simulink model "BaseEngineController_LS_128"  (Simulink 7.7)
settings: Solver=FixedStepDiscrete  StartTime=0.0  StopTime=10.0  RelTol=1e-3
PreLoadFcn:
  | try, eval([bdroot '_setup']); catch, eval('model_setup', ''); end
InitFcn:
  | try, eval([bdroot '_setup']); catch, eval('model_setup', ''); end
undefined symbols (not defined in the file): ECU565, High, motohawk_build_version, motohawk_trunc_name, motohawk_vardec_config_group, motohawk_vardec_path, True
libraries: MotoHawk_lib x1418, motohawk_control_primitives_lib x183, motohawk_engine_lib x32, simulink x21, motohawk_annotations_lib x9, AutoDoc_lib x8, simulink_extras x4, motohawk_ccp_examples_lib x1, motohawk_control_primitives_motoshare_lib x1
(part 20 of 27)

== system BaseEngineController_LS_128/Foreground/Control/Controller/Run/AC Control/AC Comp Low Pressure ==
  HiThresh : Inport
  LowThresh : Inport  Port=2
  Signal : Inport  Port=3
  Hysteresis : Subsystem
  LT : RelationalOperator  ZeroCross=off  InputSameDT=on
  LT1 : RelationalOperator  Operator=<=  ZeroCross=off  InputSameDT=on
  Threshold : Outport
  wires:
  LT/1 -> Hysteresis/1(Hi)  "AboveHiTarget"
  LT1/1 -> Hysteresis/2(Lo)  "BelowLoTarget"
  Signal/1 -> LT/1, LT1/1
  Hysteresis/1("Out (Lo=0, Hi=1)") -> Threshold/1
  HiThresh/1 -> LT/2
  LowThresh/1 -> LT1/2

== system BaseEngineController_LS_128/Foreground/Control/Controller/Run/AC Control/AC Comp Overspeed ==
  HiThresh : Inport
  LowThresh : Inport  Port=2
  Signal : Inport  Port=3
  Hysteresis : Subsystem
  LT : RelationalOperator  ZeroCross=off  InputSameDT=on
  LT1 : RelationalOperator  Operator=<=  ZeroCross=off  InputSameDT=on
  Threshold : Outport
  wires:
  LT/1 -> Hysteresis/1(Hi)  "AboveHiTarget"
  LT1/1 -> Hysteresis/2(Lo)  "BelowLoTarget"
  Signal/1 -> LT/1, LT1/1
  Hysteresis/1("Out (Lo=0, Hi=1)") -> Threshold/1
  HiThresh/1 -> LT/2
  LowThresh/1 -> LT1/2

== system BaseEngineController_LS_128/Foreground/Control/Controller/Run/AC Control/AC Comp Overspeed1 ==
  HiThresh : Inport
  LowThresh : Inport  Port=2
  Signal : Inport  Port=3
  Hysteresis : Subsystem
  LT : RelationalOperator  ZeroCross=off  InputSameDT=on
  LT1 : RelationalOperator  Operator=<=  ZeroCross=off  InputSameDT=on
  Threshold : Outport
  wires:
  LT/1 -> Hysteresis/1(Hi)  "AboveHiTarget"
  LT1/1 -> Hysteresis/2(Lo)  "BelowLoTarget"
  Signal/1 -> LT/1, LT1/1
  Hysteresis/1("Out (Lo=0, Hi=1)") -> Threshold/1
  HiThresh/1 -> LT/2
  LowThresh/1 -> LT1/2

== system BaseEngineController_LS_128/Foreground/Control/Controller/Run/AC Control/AC Comp Underspeed ==
  HiThresh : Inport
  LowThresh : Inport  Port=2
  Signal : Inport  Port=3
  Hysteresis : Subsystem
  LT : RelationalOperator  ZeroCross=off  InputSameDT=on
  LT1 : RelationalOperator  Operator=<=  ZeroCross=off  InputSameDT=on
  Threshold : Outport
  wires:
  LT/1 -> Hysteresis/1(Hi)  "AboveHiTarget"
  LT1/1 -> Hysteresis/2(Lo)  "BelowLoTarget"
  Signal/1 -> LT/1, LT1/1
  Hysteresis/1("Out (Lo=0, Hi=1)") -> Threshold/1
  HiThresh/1 -> LT/2
  LowThresh/1 -> LT1/2

== system BaseEngineController_LS_128/Foreground/Control/Controller/Run/AC Control/AC Evap Temp Hyst ==
  HiThresh : Inport
  LowThresh : Inport  Port=2
  Signal : Inport  Port=3
  Hysteresis : Subsystem
  LT : RelationalOperator  ZeroCross=off  InputSameDT=on
  LT1 : RelationalOperator  Operator=<=  ZeroCross=off  InputSameDT=on
  Threshold : Outport
  wires:
  LT/1 -> Hysteresis/1(Hi)  "AboveHiTarget"
  LT1/1 -> Hysteresis/2(Lo)  "BelowLoTarget"
  Signal/1 -> LT/1, LT1/1
  Hysteresis/1("Out (Lo=0, Hi=1)") -> Threshold/1
  HiThresh/1 -> LT/2
  LowThresh/1 -> LT1/2

== system BaseEngineController_LS_128/Foreground/Control/Controller/Run/AirFlow Manager/ShutDownTasksComplete Reset ==
  Enable : EnablePort
  Constant : Constant  Value=boolean(1)
  motohawk_data_write : MotoHawk_lib/Data Storage Blocks/motohawk_data_write  source=Lookup By Name  structure=Scalar  operation=Write entire data structure at once  sz_vec=-1  sz_row=3  sz_col=2  typ=boolean  nam='ShutDownTasksComplete'  checkNull=off  write_read_only=off  struct_inst_name='Struct1'  struct_name='MyStruct'
  wires:
  Constant/1 -> motohawk_data_write/1

== system BaseEngineController_LS_128/Foreground/Control/Controller/Run/Base Equiv Ratio/Warm Up Fuel Holdoff ==
  TimeSinceRun : Inport
  WarmuUpTimeRatio : Inport  Port=2
  ECTIdx : Inport  Port=3
  Constant : Constant
  Relational Operator : RelationalOperator  OutDataTypeStr=boolean
  Switch : Switch  Criteria=u2 > Threshold
  motohawk_interpolation_1d : MotoHawk_lib/Lookup Tables/motohawk_interpolation_1d  nam='Warmup_Time_Holdoff'  table_data=[0.1 0.1 0.1 0.1 0.1]  show_more=on  data_type=Inherit from 'Table Data'  storage=NonAdaptive  read_level=1  write_level=1  ovr_cals=on  use_help=on  help='Time before warmup fuel multiplier active'  units='sec'  use_min_max=on  min_val=0  max_val=3  use_precision=on  precision='1.3'  gain=1  offset=0  exp=1  use_links=off  prelookup_block=''  output_name=''  use_mototune_group=off  mototune_group=motohawk_vardec_path(gcb)
  Out1 : Outport
  wires:
  ECTIdx/1 -> motohawk_interpolation_1d/1
  motohawk_interpolation_1d/1 -> Relational Operator/2
  TimeSinceRun/1 -> Relational Operator/1
  Relational Operator/1 -> Switch/2
  WarmuUpTimeRatio/1 -> Switch/1
  Constant/1 -> Switch/3
  Switch/1 -> Out1/1

== system BaseEngineController_LS_128/Foreground/Control/Controller/Run/Boost Control/BoostControl Adapt ==
  Active State : Inport
  ITerm : Inport  Port=2
  Enable : EnablePort
  Abs : Abs  SaturateOnIntegerOverflow=on
  Adapt Boost Table : Subsystem  TreatAsAtomicUnit=on
  BoostControl Enable Delay : Subsystem  TreatAsAtomicUnit=on
  Logical Operator1 : Logic  Inputs=3
  Product0 : Product  SaturateOnIntegerOverflow=on  InputSameDT=on  OutDataTypeStr=Inherit: Same as first input
  Relational Operator : RelationalOperator  Operator=<=  InputSameDT=on
  Saturation (Tunable) : Subsystem  AncestorBlock=motohawk_control_primitives_lib/Saturation (Tunable)  mask(Saturation (Tunable)){prefix='BoostAdaptError', UprLim=1, LwrLim=-1, units='', grp=motohawk_vardec_path(gcb)}
      mask prompts: UprLim "Upper Limit"; LwrLim "Lower Limit"; grp "MotoTune Group String"
      mask help: Saturation block with calibratable min/max values.
      mask Display:
      | patch([0 0 1 1], [0 0.075 0.075 0], [230/255 0/255 0/255])
      | patch([0 0 1 1], [0.025 0.05 0.05 0.025], [150/255 0/255 0/255])
      | patch([0 0 1 1], [0 0.025 0.025 0], [0/255 0/255 0/255])
      | 
      | plot([0 .2 .8 1], [.1 .1 1 1])
  motohawk_calibration2 : MotoHawk_lib/Calibration & Probing Blocks/motohawk_calibration  nam='BoostControlAdaptGain'  val=0.001  storage=Calibration  show_more=on  name_source=Use Parameter  data_type=Inherit from 'Default Value'  read_level=1  write_level=1  ovr_cals=on  view_as=Number  enum_struct={'Disabled', 'Enabled'}  vector_style=Wide Row  use_help_units=off  help="'Gain for updating BaseAirflow table.  This fraction of the error is added to the map every 5ms.'"  units='mult'  use_header_enum=off  row_header_enum={}  col_header_enum={}  use_min_max=off  min_val=-inf  max_val=inf  use_precision=on  precision='1.4'  gain=1  offset=0  exp=1  use_mototune_group=on  mototune_group=motohawk_vardec_path(gcb)
  motohawk_calibration3 : MotoHawk_lib/Calibration & Probing Blocks/motohawk_calibration  nam='BoostControlAdaptDelta'  val=2  storage=Calibration  show_more=on  name_source=Use Parameter  data_type=Inherit from 'Default Value'  read_level=1  write_level=1  ovr_cals=on  view_as=Number  enum_struct={'Disabled', 'Enabled'}  vector_style=Wide Row  use_help_units=on  help='Air PID Iterm must be less than this delta to adapt the BaseAirflow table.'  units='mult'  use_header_enum=off  row_header_enum={}  col_header_enum={}  use_min_max=on  min_val=-inf  max_val=inf  use_precision=off  precision=''  gain=1  offset=0  exp=1  use_mototune_group=on  mototune_group=motohawk_vardec_path(gcb)
  motohawk_calibration4 : MotoHawk_lib/Calibration & Probing Blocks/motohawk_calibration  nam='BoostControlAdaptEnable'  val=false  storage=Calibration  show_more=on  name_source=Use Parameter  data_type=Inherit from 'Default Value'  read_level=1  write_level=1  ovr_cals=on  view_as=Enumeration  enum_struct={'Disabled', 'Enabled'}  vector_style=Wide Row  use_help_units=on  help='Determines whether the BaseAirflow table will be adapted using the air PID Iterm.'  units='bool'  use_header_enum=off  row_header_enum={}  col_header_enum={}  use_min_max=off  min_val=-inf  max_val=inf  use_precision=off  precision=''  gain=1  offset=0  exp=1  use_mototune_group=on  mototune_group=motohawk_vardec_path(gcb)
  motohawk_probe3 : MotoHawk_lib/Calibration & Probing Blocks/motohawk_probe  nam='BoostControlAdaptEnabled'  show_more=on  name_source=Use Parameter  read_level=1  view_as=Enumeration  enum_struct={'Not Enabled', 'Enabled'}  vector_style=Wide Row  use_help_units=on  help=''  units=''  use_header_enum=off  row_header_enum={}  col_header_enum={}  use_precision=off  precision=''  gain=1  offset=0  exp=1  use_mototune_group=on  mototune_group=motohawk_vardec_path(gcb)
  wires:
  Abs/1 -> Relational Operator/1
  motohawk_calibration3/1 -> Relational Operator/2
  motohawk_calibration2/1 -> Product0/2
  Product0/1 -> Saturation (Tunable)/1(In)
  ITerm/1 -> Product0/1, Abs/1
  Relational Operator/1 -> Logical Operator1/3
  BoostControl Enable Delay/1(State_Out) -> Logical Operator1/2
  Logical Operator1/1 -> motohawk_probe3/1, Adapt Boost Table/Enable
  Saturation (Tunable)/1(Out) -> Adapt Boost Table/1(error)
  motohawk_calibration4/1 -> Logical Operator1/1
  Active State/1 -> BoostControl Enable Delay/1(State_In)

== system BaseEngineController_LS_128/Foreground/Control/Controller/Run/Boost Control/Universal PID (Tunable & Scheduled) ==
  Actual : Inport
  SetPoint : Inport  Port=2
  ResetAll : Inport  Port=3
  Constant : Constant  Value=0  OutDataTypeStr=Inherit: Inherit via back propagation
  Constant1 : Constant  Value=0
  PID Gain Select1 : Subsystem
  Saturation : motohawk_control_primitives_lib/Saturation  SystemSampleTime=-1
  Switch : Switch  Threshold=0.5
  Universal PID : motohawk_control_primitives_lib/Universal PID  Description=|  SystemSampleTime=-1  samp_time=.005
      | /* Name: ErrorGain Unit:mult ClassID:VAR StorageID:FLASH Access:RW4+RW3+NA2+NA1 TypeID:UINT4                   
      |    Gain:0.000000001 Min:0.000000000 Max:4.000000000 Format:10.9 UpdateID:REMOTE Help:"This gain is applied to "
      |    "the error term before it is used to calculate the P, I and D terms." VardecSig:6C */                       
      |                                                                                                                
      | /* Name: ITermLowerLim Unit:0 ClassID:VAR StorageID:FLASH Access:RW4+RW3+NA2+NA1 TypeID:SINT2 Gain:0.1         
      |    Min:-3276.8 Max:3276.7 Format:5.1 UpdateID:REMOTE Help:"Lower limit on the I-term value." VardecSig:6C */   
      |                                                                                                                
      | /* Name: ITermUpperLim ClassID:VAR StorageID:FLASH Access:RW4+RW3+NA2+NA1 TypeID:SINT2 Gain:0.1 Min:-3276.8    
      |    Max:3276.7 Format:5.1 UpdateID:REMOTE Help:"Upper limit on I-term value." VardecSig:6C */                   
      |                                                                                                                
      | /* Name: PIDOutLowerLim ClassID:VAR StorageID:FLASH Access:RW4+RW3+NA2+NA1 TypeID:SINT2 Gain:0.1               
      |    Min:-3276.8 Max:3276.7 Format:5.1 UpdateID:REMOTE Help:"Lower limit on PID output." VardecSig:6C */         
      |                                                                                                                
      | /* Name: PIDOutUpperLim ClassID:VAR StorageID:FLASH Access:RW4+RW3+NA2+NA1 TypeID:SINT2 Gain:0.1               
      |    Min:-3276.8 Max:3276.7 Format:3.1 UpdateID:REMOTE Help:"Upper limit on PID output." VardecSig:6C */
  motohawk_calibration2 : MotoHawk_lib/Calibration & Probing Blocks/motohawk_calibration  nam=[prefix 'PIDOutUpperLimit']  val=150  storage=Calibration  show_more=on  name_source=Use Parameter  data_type=Inherit from 'Default Value'  read_level=1  write_level=1  ovr_cals=on  view_as=Number  enum_struct={'Disabled', 'Enabled'}  vector_style=Wide Row  use_help_units=on  help='Upper limit on air min governor PID Output.'  units=units  use_header_enum=off  row_header_enum={}  col_header_enum={}  use_min_max=off  min_val=-inf  max_val=inf  use_precision=off  precision=''  gain=1  offset=0  exp=1  use_mototune_group=on  mototune_group=[group ' | Air PID Config']
  motohawk_calibration5 : MotoHawk_lib/Calibration & Probing Blocks/motohawk_calibration  nam=[prefix 'ErrorGain']  val=0.4  storage=Calibration  show_more=on  name_source=Use Parameter  data_type=Inherit from 'Default Value'  read_level=1  write_level=1  ovr_cals=on  view_as=Number  enum_struct={'Disabled', 'Enabled'}  vector_style=Wide Row  use_help_units=on  help='Error gain for the min governor controller. This gain is applied to the RPM error term before it is used to calculate the P, I and D terms.'  units='mult'  use_header_enum=off  row_header_enum={}  col_header_enum={}  use_min_max=on  min_val=-inf  max_val=inf  use_precision=off  precision=''  gain=1  offset=0  exp=1  use_mototune_group=on  mototune_group=[group ' | Air PID Config']
  motohawk_calibration7 : MotoHawk_lib/Calibration & Probing Blocks/motohawk_calibration  nam=[prefix 'ITermLowerLimit']  val=-3  storage=Calibration  show_more=on  name_source=Use Parameter  data_type=Inherit from 'Default Value'  read_level=1  write_level=1  ovr_cals=on  view_as=Number  enum_struct={'Disabled', 'Enabled'}  vector_style=Wide Row  use_help_units=on  help='Lower limit on Air Min Governor I-term value.'  units=units  use_header_enum=off  row_header_enum={}  col_header_enum={}  use_min_max=on  min_val=-inf  max_val=inf  use_precision=off  precision=''  gain=1  offset=0  exp=1  use_mototune_group=on  mototune_group=[group ' | Air PID Config']
  motohawk_calibration8 : MotoHawk_lib/Calibration & Probing Blocks/motohawk_calibration  nam=[prefix 'ITermUpperLimit']  val=55  storage=Calibration  show_more=on  name_source=Use Parameter  data_type=Inherit from 'Default Value'  read_level=1  write_level=1  ovr_cals=on  view_as=Number  enum_struct={'Disabled', 'Enabled'}  vector_style=Wide Row  use_help_units=on  help='Upper limit on Air Min Governor I-term value.'  units=units  use_header_enum=off  row_header_enum={}  col_header_enum={}  use_min_max=on  min_val=-inf  max_val=inf  use_precision=off  precision=''  gain=1  offset=0  exp=1  use_mototune_group=on  mototune_group=[group ' | Air PID Config']
  motohawk_calibration9 : MotoHawk_lib/Calibration & Probing Blocks/motohawk_calibration  nam=[prefix 'PIDOutLowerLimit']  val=-10  storage=Calibration  show_more=on  name_source=Use Parameter  data_type=Inherit from 'Default Value'  read_level=1  write_level=1  ovr_cals=on  view_as=Number  enum_struct={'Disabled', 'Enabled'}  vector_style=Wide Row  use_help_units=on  help='Lower limit on air min governor PID Output.'  units=units  use_header_enum=off  row_header_enum={}  col_header_enum={}  use_min_max=on  min_val=-inf  max_val=inf  use_precision=off  precision=''  gain=1  offset=0  exp=1  use_mototune_group=on  mototune_group=[group ' | Air PID Config']
  motohawk_prelookup1 : MotoHawk_lib/Lookup Tables/motohawk_prelookup  nam=[prefix 'SpeedError']  breakpoint_data=[-200 -90 -30 0 50 103 140 177 213]  show_more=on  data_type=Inherit from 'Table Data'  storage=Constant  read_level=1  write_level=1  ovr_cals=on  use_help=on  help=''  units=''  use_min_max=off  min_val=-inf  max_val=inf  use_precision=off  precision=''  gain=1  offset=0  exp=1  use_links=off  input_name=''  use_mototune_group=on  mototune_group=motohawk_vardec_path(gcb)
  motohawk_probe1 : MotoHawk_lib/Calibration & Probing Blocks/motohawk_probe  nam=[prefix 'PTerm']  show_more=on  name_source=Use Parameter  read_level=1  view_as=Number  enum_struct={'Disabled', 'Enabled'}  vector_style=Wide Row  use_help_units=on  help='Air min governor P term'  units=''  use_header_enum=off  row_header_enum={}  col_header_enum={}  use_precision=on  precision=''  gain=1  offset=0  exp=1  use_mototune_group=on  mototune_group=motohawk_vardec_path(gcb)
  motohawk_probe2 : MotoHawk_lib/Calibration & Probing Blocks/motohawk_probe  nam=[prefix 'ITerm']  show_more=on  name_source=Use Parameter  read_level=1  view_as=Number  enum_struct={'Disabled', 'Enabled'}  vector_style=Wide Row  use_help_units=on  help='Air min governor I term'  units=''  use_header_enum=off  row_header_enum={}  col_header_enum={}  use_precision=on  precision=''  gain=1  offset=0  exp=1  use_mototune_group=on  mototune_group=motohawk_vardec_path(gcb)
  motohawk_probe3 : MotoHawk_lib/Calibration & Probing Blocks/motohawk_probe  nam=[prefix 'DTerm']  show_more=on  name_source=Use Parameter  read_level=1  view_as=Number  enum_struct={'Disabled', 'Enabled'}  vector_style=Wide Row  use_help_units=on  help='Air min governor D term'  units=''  use_header_enum=off  row_header_enum={}  col_header_enum={}  use_precision=on  precision=''  gain=1  offset=0  exp=1  use_mototune_group=on  mototune_group=motohawk_vardec_path(gcb)
  motohawk_probe6 : MotoHawk_lib/Calibration & Probing Blocks/motohawk_probe  nam=[prefix 'Error']  show_more=on  name_source=Use Parameter  read_level=1  view_as=Number  enum_struct={'Disabled', 'Enabled'}  vector_style=Wide Row  use_help_units=on  help='Air min governor P term'  units=''  use_header_enum=off  row_header_enum={}  col_header_enum={}  use_precision=on  precision=''  gain=1  offset=0  exp=1  use_mototune_group=on  mototune_group=motohawk_vardec_path(gcb)
  MinGovOut : Outport
  MinGovITerm : Outport  Port=2
  wires:
  motohawk_prelookup1/1 -> PID Gain Select1/1(ErrorIdx)
  PID Gain Select1/3(DGain) -> Universal PID/6
  PID Gain Select1/1(PGain) -> Universal PID/4
  motohawk_calibration5/1 -> Universal PID/3
  Universal PID/1 -> Saturation/1
  Universal PID/5 -> motohawk_probe3/1
  Actual/1 -> Universal PID/1
  SetPoint/1 -> Universal PID/2
  PID Gain Select1/2(IGain) -> Universal PID/5
  Universal PID/2 -> motohawk_prelookup1/1, motohawk_probe6/1
  Universal PID/3 -> motohawk_probe1/1
  Universal PID/4 -> motohawk_probe2/1, MinGovITerm/1
  ResetAll/1 -> Universal PID/10, Switch/2
  Constant/1 -> Universal PID/7
  motohawk_calibration7/1 -> Universal PID/8
  motohawk_calibration8/1 -> Universal PID/9
  motohawk_calibration2/1 -> Saturation/3
  motohawk_calibration9/1 -> Saturation/2
  Constant1/1 -> Switch/1
  Saturation/1 -> Switch/3
  Switch/1 -> MinGovOut/1

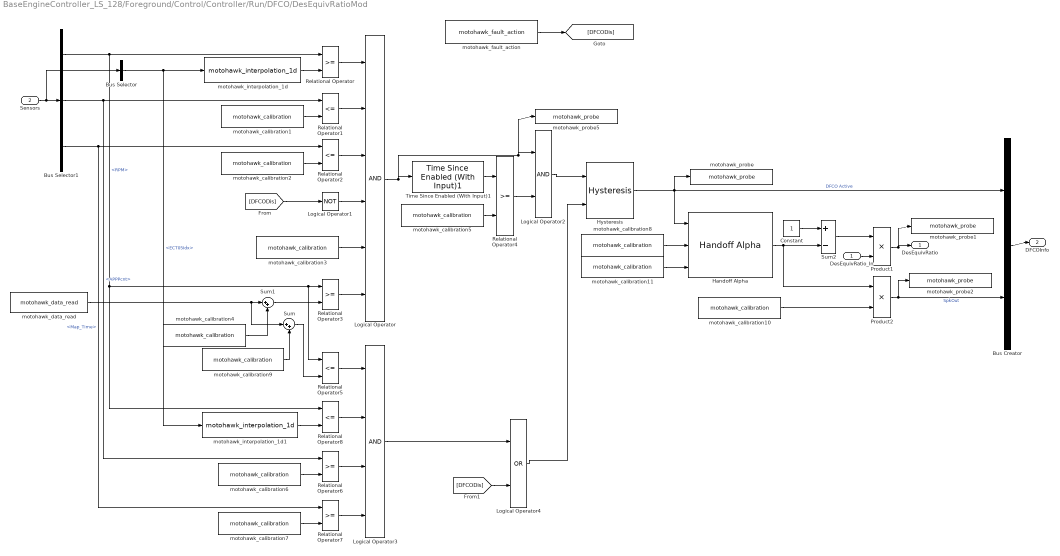
== system BaseEngineController_LS_128/Foreground/Control/Controller/Run/DFCO/DesEquivRatioMod ==
  DesEquivRatio_In : Inport
  Sensors : Inport  Port=2
  Bus Creator : BusCreator  Inputs=2
  Bus Selector : BusSelector  OutputSignals=RawIndexes.ECT05Idx
  Bus Selector1 : BusSelector  OutputSignals=Raw.RPM,RawProcessed.APPPcnt,Raw.LinearSensors.Map_Time
  Constant : Constant
  Handoff Alpha : motohawk_control_primitives_lib/Handoff Alpha  SystemSampleTime=-1  samp_time=-1
  Hysteresis : motohawk_control_primitives_lib/Hysterisis/Hysteresis  SystemSampleTime=-1
  Logical Operator : Logic  Inputs=6  AllPortsSameDT=off  OutDataTypeStr=boolean
  Logical Operator1 : Logic  Operator=NOT  Inputs=5  AllPortsSameDT=off  OutDataTypeStr=boolean
  Logical Operator2 : Logic  AllPortsSameDT=off  OutDataTypeStr=boolean
  Logical Operator3 : Logic  Inputs=4  AllPortsSameDT=off  OutDataTypeStr=boolean
  Logical Operator4 : Logic  Operator=OR  AllPortsSameDT=off  OutDataTypeStr=boolean
  Product1 : Product  RndMeth=Zero
  Product2 : Product  RndMeth=Zero
  Relational Operator{,3..4,6..7} (5 alike) : RelationalOperator  OutDataTypeStr=boolean
  Relational Operator{1..2,5,8} (4 alike) : RelationalOperator  Operator=<=  OutDataTypeStr=boolean
  Sum : Sum  Inputs=|++
  Sum1 : Sum  Inputs=|++
  Sum2 : Sum  Inputs=+-
  Time Since Enabled (With Input)1 : motohawk_control_primitives_lib/Time Since Enabled (With Input)1  SystemSampleTime=-1  nam='DFCOEnterTimer'  samp_time=-1  init=0  upperlim=16000
  motohawk_calibration1 : MotoHawk_lib/Calibration & Probing Blocks/motohawk_calibration  nam='DFCOEntryAPP'  val=2  storage=Calibration  show_more=on  name_source=Use Parameter  data_type=Inherit from 'Default Value'  read_level=1  write_level=1  ovr_cals=on  view_as=Number  enum_struct={'Disabled', 'Enabled'}  vector_style=Wide Row  use_help_units=on  help='DFCO APP entry threshold'  units='%'  use_header_enum=off  row_header_enum={}  col_header_enum={}  use_min_max=on  min_val=0  max_val=100  use_precision=off  precision=''  gain=1  offset=0  exp=1  use_mototune_group=off  mototune_group=motohawk_vardec_path(gcb)
  motohawk_calibration10 : MotoHawk_lib/Calibration & Probing Blocks/motohawk_calibration  nam='DFCOExitSparkRet'  val=-10  storage=Calibration  show_more=on  name_source=Use Parameter  data_type=int16  read_level=1  write_level=1  ovr_cals=on  view_as=Number  enum_struct={'Disabled', 'Enabled'}  vector_style=Wide Row  use_help_units=on  help='DFCO exit spark retard'  units='degBTDC'  use_header_enum=off  row_header_enum={}  col_header_enum={}  use_min_max=on  min_val=-100  max_val=100  use_precision=off  precision=''  gain=1  offset=0  exp=1  use_mototune_group=off  mototune_group=motohawk_vardec_path(gcb)
  motohawk_calibration11 : MotoHawk_lib/Calibration & Probing Blocks/motohawk_calibration  nam='DFCOExitRampTime'  val=.5  storage=Calibration  show_more=on  name_source=Use Parameter  data_type=Inherit from 'Default Value'  read_level=1  write_level=1  ovr_cals=on  view_as=Number  enum_struct={'Disabled', 'Enabled'}  vector_style=Wide Row  use_help_units=on  help='DFCO exit ramp time'  units='sec'  use_header_enum=off  row_header_enum={}  col_header_enum={}  use_min_max=off  min_val=-inf  max_val=inf  use_precision=off  precision=''  gain=1  offset=0  exp=1  use_mototune_group=off  mototune_group=motohawk_vardec_path(gcb)
  motohawk_calibration2 : MotoHawk_lib/Calibration & Probing Blocks/motohawk_calibration  nam='DFCOEntryMAP'  val=28  storage=Calibration  show_more=on  name_source=Use Parameter  data_type=uint8  read_level=1  write_level=1  ovr_cals=on  view_as=Number  enum_struct={'Disabled', 'Enabled'}  vector_style=Wide Row  use_help_units=on  help='DFCO MAP entry threshold'  units='kPa'  use_header_enum=off  row_header_enum={}  col_header_enum={}  use_min_max=on  min_val=0  max_val=1000  use_precision=off  precision=''  gain=1  offset=0  exp=1  use_mototune_group=off  mototune_group=motohawk_vardec_path(gcb)
  motohawk_calibration3 : MotoHawk_lib/Calibration & Probing Blocks/motohawk_calibration  nam='DFCOEnable'  val=0  storage=Calibration  show_more=on  name_source=Use Parameter  data_type=boolean  read_level=1  write_level=1  ovr_cals=on  view_as=Enumeration  enum_struct={'Disabled', 'Enabled'}  vector_style=Wide Row  use_help_units=off  help=''  units=''  use_header_enum=off  row_header_enum={}  col_header_enum={}  use_min_max=off  min_val=-inf  max_val=inf  use_precision=off  precision=''  gain=1  offset=0  exp=1  use_mototune_group=off  mototune_group=motohawk_vardec_path(gcb)
  motohawk_calibration4 : MotoHawk_lib/Calibration & Probing Blocks/motohawk_calibration  nam='DFCOEnterIdleSpeed'  val=300  storage=Calibration  show_more=on  name_source=Use Parameter  data_type=int16  read_level=1  write_level=1  ovr_cals=on  view_as=Number  enum_struct={'Disabled', 'Enabled'}  vector_style=Wide Row  use_help_units=on  help='DFCO entry above idle speed setpoint'  units='RPM'  use_header_enum=off  row_header_enum={}  col_header_enum={}  use_min_max=on  min_val=0  max_val=7000  use_precision=off  precision=''  gain=1  offset=0  exp=1  use_mototune_group=off  mototune_group=motohawk_vardec_path(gcb)
  motohawk_calibration5 : MotoHawk_lib/Calibration & Probing Blocks/motohawk_calibration  nam='DFCODelayTime'  val=.6  storage=Calibration  show_more=on  name_source=Use Parameter  data_type=Inherit from 'Default Value'  read_level=1  write_level=1  ovr_cals=on  view_as=Number  enum_struct={'Disabled', 'Enabled'}  vector_style=Wide Row  use_help_units=on  help='DFCO delay enter time'  units='sec'  use_header_enum=off  row_header_enum={}  col_header_enum={}  use_min_max=on  min_val=0  max_val=1000000  use_precision=off  precision=''  gain=1  offset=0  exp=1  use_mototune_group=off  mototune_group=motohawk_vardec_path(gcb)
  motohawk_calibration6 : MotoHawk_lib/Calibration & Probing Blocks/motohawk_calibration  nam='DFCOExitAPP'  val=4  storage=Calibration  show_more=on  name_source=Use Parameter  data_type=Inherit from 'Default Value'  read_level=1  write_level=1  ovr_cals=on  view_as=Number  enum_struct={'Disabled', 'Enabled'}  vector_style=Wide Row  use_help_units=on  help='DFCO exit APP threshold'  units='%'  use_header_enum=off  row_header_enum={}  col_header_enum={}  use_min_max=on  min_val=0  max_val=100  use_precision=off  precision=''  gain=1  offset=0  exp=1  use_mototune_group=off  mototune_group=motohawk_vardec_path(gcb)
  motohawk_calibration7 : MotoHawk_lib/Calibration & Probing Blocks/motohawk_calibration  nam='DFCOExitMAP'  val=50  storage=Calibration  show_more=on  name_source=Use Parameter  data_type=uint8  read_level=1  write_level=1  ovr_cals=on  view_as=Number  enum_struct={'Disabled', 'Enabled'}  vector_style=Wide Row  use_help_units=on  help='DFCO exit MAP threhsold'  units='kPa'  use_header_enum=off  row_header_enum={}  col_header_enum={}  use_min_max=on  min_val=0  max_val=1000  use_precision=off  precision=''  gain=1  offset=0  exp=1  use_mototune_group=off  mototune_group=motohawk_vardec_path(gcb)
  motohawk_calibration8 : MotoHawk_lib/Calibration & Probing Blocks/motohawk_calibration  nam='DFCOEnterRampTime'  val=.5  storage=Calibration  show_more=on  name_source=Use Parameter  data_type=Inherit from 'Default Value'  read_level=1  write_level=1  ovr_cals=on  view_as=Number  enum_struct={'Disabled', 'Enabled'}  vector_style=Wide Row  use_help_units=on  help='DFCO enter ramp time'  units='sec'  use_header_enum=off  row_header_enum={}  col_header_enum={}  use_min_max=off  min_val=-inf  max_val=inf  use_precision=off  precision=''  gain=1  offset=0  exp=1  use_mototune_group=off  mototune_group=motohawk_vardec_path(gcb)
  motohawk_calibration9 : MotoHawk_lib/Calibration & Probing Blocks/motohawk_calibration  nam='DFCOExitIdleSpeed'  val=100  storage=Calibration  show_more=on  name_source=Use Parameter  data_type=int16  read_level=1  write_level=1  ovr_cals=on  view_as=Number  enum_struct={'Disabled', 'Enabled'}  vector_style=Wide Row  use_help_units=on  help='DFCO exit offset from desired idle speed'  units='RPM'  use_header_enum=off  row_header_enum={}  col_header_enum={}  use_min_max=on  min_val=0  max_val=7000  use_precision=off  precision=''  gain=1  offset=0  exp=1  use_mototune_group=off  mototune_group=motohawk_vardec_path(gcb)
  motohawk_data_read : MotoHawk_lib/Data Storage Blocks/motohawk_data_read  source=Lookup By Name  structure=Scalar  operation=Read scalar from location by index  sz_vec=4  sz_row=2  sz_col=3  typ=double  nam='MinGovRPMSetPt'  checkNull=on  struct_inst_name='MyData'  struct_nam='MyStruct'
  motohawk_fault_action : MotoHawk_lib/Fault Management Blocks/motohawk_fault_action  nam='DFCODisable'  output_status=on  eval_nam=DFCODisable
  motohawk_interpolation_1d : MotoHawk_lib/Lookup Tables/motohawk_interpolation_1d  nam='DFCOEntryRPM'  table_data=[0 0 0 0 0]  show_more=off  data_type=Inherit from 'Table Data'  storage=NonAdaptive  read_level=1  write_level=1  ovr_cals=on  use_help=off  help=''  units=''  use_min_max=off  min_val=-inf  max_val=inf  use_precision=off  precision=''  gain=1  offset=0  exp=1  use_links=off  prelookup_block=''  output_name=''  use_mototune_group=off  mototune_group=motohawk_vardec_path(gcb)
  motohawk_interpolation_1d1 : MotoHawk_lib/Lookup Tables/motohawk_interpolation_1d  nam='DFCOExitRPM'  table_data=[0 0 0 0 0]  show_more=off  data_type=Inherit from 'Table Data'  storage=NonAdaptive  read_level=1  write_level=1  ovr_cals=on  use_help=off  help=''  units=''  use_min_max=off  min_val=-inf  max_val=inf  use_precision=off  precision=''  gain=1  offset=0  exp=1  use_links=off  prelookup_block=''  output_name=''  use_mototune_group=off  mototune_group=motohawk_vardec_path(gcb)
  motohawk_probe : MotoHawk_lib/Calibration & Probing Blocks/motohawk_probe  nam='DFCOActive'  show_more=on  name_source=Use Parameter  read_level=1  view_as=Number  enum_struct={'Disabled', 'Enabled'}  vector_style=Wide Row  use_help_units=on  help='DFCO state'  units=''  use_header_enum=off  row_header_enum={}  col_header_enum={}  use_precision=off  precision=''  gain=1  offset=0  exp=1  use_mototune_group=off  mototune_group=motohawk_vardec_path(gcb)
  motohawk_probe1 : MotoHawk_lib/Calibration & Probing Blocks/motohawk_probe  nam='DFCODesEquivRatio'  show_more=on  name_source=Use Parameter  read_level=1  view_as=Number  enum_struct={'Disabled', 'Enabled'}  vector_style=Wide Row  use_help_units=on  help='DFCO commanded equiv ratio'  units=''  use_header_enum=off  row_header_enum={}  col_header_enum={}  use_precision=off  precision=''  gain=1  offset=0  exp=1  use_mototune_group=off  mototune_group=motohawk_vardec_path(gcb)
  motohawk_probe2 : MotoHawk_lib/Calibration & Probing Blocks/motohawk_probe  nam='DFCODesSparkOutOfst'  show_more=on  name_source=Use Parameter  read_level=1  view_as=Number  enum_struct={'Disabled', 'Enabled'}  vector_style=Wide Row  use_help_units=on  help='DFCO spark output'  units='degBTDC'  use_header_enum=off  row_header_enum={}  col_header_enum={}  use_precision=off  precision=''  gain=1  offset=0  exp=1  use_mototune_group=off  mototune_group=motohawk_vardec_path(gcb)
  motohawk_probe5 : MotoHawk_lib/Calibration & Probing Blocks/motohawk_probe  nam='DFCOEnterCond'  show_more=on  name_source=Use Parameter  read_level=1  view_as=Number  enum_struct={'Disabled', 'Enabled'}  vector_style=Wide Row  use_help_units=on  help='Conditions are correct for DFCO'  units=''  use_header_enum=off  row_header_enum={}  col_header_enum={}  use_precision=off  precision=''  gain=1  offset=0  exp=1  use_mototune_group=off  mototune_group=motohawk_vardec_path(gcb)
  DesEquivRatio : Outport
  DFCOInfo : Outport  Port=2
  wires:
  Sensors/1 -> Bus Selector1/1, Bus Selector/1
  Bus Selector1/1 -> Relational Operator/1, Relational Operator8/1, Relational Operator3/1, Relational Operator5/1  "<RPM>"
  motohawk_calibration1/1 -> Relational Operator1/2
  Bus Selector1/2 -> Relational Operator1/1, Relational Operator6/1  "<APPPcnt>"
  motohawk_calibration2/1 -> Relational Operator2/2
  Bus Selector1/3 -> Relational Operator2/1, Relational Operator7/1  "<Map_Time>"
  motohawk_fault_action/1 -> [DFCODis]
  Relational Operator/1 -> Logical Operator/1
  Relational Operator1/1 -> Logical Operator/2
  Relational Operator2/1 -> Logical Operator/3
  Logical Operator1/1 -> Logical Operator/4
  motohawk_calibration3/1 -> Logical Operator/5
  Relational Operator3/1 -> Logical Operator/6
  Logical Operator/1 -> Time Since Enabled (With Input)1/1, Logical Operator2/1, motohawk_probe5/1
  Time Since Enabled (With Input)1/1 -> Relational Operator4/1
  motohawk_calibration5/1 -> Relational Operator4/2
  Relational Operator4/1 -> Logical Operator2/2
  motohawk_calibration6/1 -> Relational Operator6/2
  motohawk_calibration7/1 -> Relational Operator7/2
  Relational Operator5/1 -> Logical Operator3/1
  Relational Operator8/1 -> Logical Operator3/2
  Relational Operator7/1 -> Logical Operator3/4
  Relational Operator6/1 -> Logical Operator3/3
  Logical Operator2/1 -> Hysteresis/1
  motohawk_calibration4/1 -> Sum1/2
  motohawk_calibration9/1 -> Sum/2
  Hysteresis/1 -> Bus Creator/1, motohawk_probe/1, Handoff Alpha/1  "DFCO Active"
  Bus Creator/1 -> DFCOInfo/1
  motohawk_data_read/1 -> Sum1/1, Sum/1
  motohawk_interpolation_1d/1 -> Relational Operator/2
  Bus Selector/1 -> motohawk_interpolation_1d/1, motohawk_interpolation_1d1/1  "<ECT05Idx>"
  motohawk_interpolation_1d1/1 -> Relational Operator8/2
  Sum1/1 -> Relational Operator3/2
  Sum/1 -> Relational Operator5/2
  Product1/1 -> DesEquivRatio/1, motohawk_probe1/1
  Product2/1 -> motohawk_probe2/1, Bus Creator/2  "SpkOut"
  Handoff Alpha/1 -> Product2/1, Sum2/2
  DesEquivRatio_In/1 -> Product1/2
  motohawk_calibration10/1 -> Product2/2
  Sum2/1 -> Product1/1
  motohawk_calibration11/1 -> Handoff Alpha/3
  motohawk_calibration8/1 -> Handoff Alpha/2
  Constant/1 -> Sum2/1
  Logical Operator3/1 -> Logical Operator4/1
  Logical Operator4/1 -> Hysteresis/2
  [DFCODis] -> Logical Operator4/2
  [DFCODis] -> Logical Operator1/1

== system BaseEngineController_LS_128/Foreground/Control/Controller/Run/FAN Control/Hysterisis ==
  HiThresh : Inport
  LowThresh : Inport  Port=2
  Signal : Inport  Port=3
  Hysteresis : Subsystem
  LT : RelationalOperator  ZeroCross=off  InputSameDT=on
  LT1 : RelationalOperator  Operator=<=  ZeroCross=off  InputSameDT=on
  Threshold : Outport
  wires:
  LT/1 -> Hysteresis/1(Hi)  "AboveHiTarget"
  LT1/1 -> Hysteresis/2(Lo)  "BelowLoTarget"
  Signal/1 -> LT/1, LT1/1
  Hysteresis/1("Out (Lo=0, Hi=1)") -> Threshold/1
  HiThresh/1 -> LT/2
  LowThresh/1 -> LT1/2

== system BaseEngineController_LS_128/Foreground/Control/Controller/Run/FAN Control/Hysterisis1 ==
  HiThresh : Inport
  LowThresh : Inport  Port=2
  Signal : Inport  Port=3
  Hysteresis : Subsystem
  LT : RelationalOperator  ZeroCross=off  InputSameDT=on
  LT1 : RelationalOperator  Operator=<=  ZeroCross=off  InputSameDT=on
  Threshold : Outport
  wires:
  LT/1 -> Hysteresis/1(Hi)  "AboveHiTarget"
  LT1/1 -> Hysteresis/2(Lo)  "BelowLoTarget"
  Signal/1 -> LT/1, LT1/1
  Hysteresis/1("Out (Lo=0, Hi=1)") -> Threshold/1
  HiThresh/1 -> LT/2
  LowThresh/1 -> LT1/2

== system BaseEngineController_LS_128/Foreground/Control/Controller/Run/FAN Control/Hysterisis2 ==
  HiThresh : Inport
  LowThresh : Inport  Port=2
  Signal : Inport  Port=3
  Hysteresis : Subsystem
  LT : RelationalOperator  ZeroCross=off  InputSameDT=on
  LT1 : RelationalOperator  Operator=<=  ZeroCross=off  InputSameDT=on
  Threshold : Outport
  wires:
  LT/1 -> Hysteresis/1(Hi)  "AboveHiTarget"
  LT1/1 -> Hysteresis/2(Lo)  "BelowLoTarget"
  Signal/1 -> LT/1, LT1/1
  Hysteresis/1("Out (Lo=0, Hi=1)") -> Threshold/1
  HiThresh/1 -> LT/2
  LowThresh/1 -> LT1/2

== system BaseEngineController_LS_128/Foreground/Control/Controller/Run/Fuel System Manager/DesiredFuelCalc ==
  FPC : Inport
  BankCals : Inport  Port=2
  BankAMult : Inport  Port=3
  BankBMult : Inport  Port=4
  Logical Operator : Logic  Operator=NOT  AllPortsSameDT=off  OutDataTypeStr=boolean
  Product : Product  RndMeth=Zero
  Product1 : Product  RndMeth=Zero
  Product2 : Product  Inputs=3  RndMeth=Zero
  DesiredFuel : Outport
  wires:
  BankAMult/1 -> Product/1
  BankCals/1 -> Product1/1, Logical Operator/1
  BankBMult/1 -> Product1/2
  Logical Operator/1 -> Product/2
  Product/1 -> Product2/2
  Product1/1 -> Product2/3
  FPC/1 -> Product2/1
  Product2/1 -> DesiredFuel/1

== system BaseEngineController_LS_128/Foreground/Control/Controller/Run/Fuel System Manager/Fuel Calculation ==
  Sensors : Inport
  O2Info : Inport  Port=2
  "Apply Multipliers for O2, Knock Control, and Enrichment1" : Product  SaturateOnIntegerOverflow=on  InputSameDT=on  OutDataTypeStr=Inherit: Same as first input
  Bus Selector : BusSelector  OutputSignals=O2FuelMult
  Bus Selector1 : BusSelector  OutputSignals=DesiredLambda.DesEquivRatio
  Calculate Fuel Flow : Subsystem
  Data Type Conversion : DataTypeConversion  SaturateOnIntegerOverflow=on  RndMeth=Zero
  Number of Combustion Events Per Revolution : MotoHawk_lib/Data Storage Blocks/motohawk_data_read  source=Lookup By Name  structure=Scalar  operation=Read scalar from location by index  sz_vec=-1  sz_row=-1  sz_col=-1  typ=uint8  nam='CombEventsPerRev'  checkNull=on  struct_inst_name='Struct1'  struct_nam='MyStruct'
  Per-Cylinder Mass Flow Rate : Product  Inputs=*/  SaturateOnIntegerOverflow=on  InputSameDT=on  OutDataTypeStr=Inherit: Same as first input
  motohawk_probe : MotoHawk_lib/Calibration & Probing Blocks/motohawk_probe  nam='GlobalBaseFuelRate'  show_more=on  name_source=Use Parameter  read_level=1  view_as=Number  enum_struct={'Disabled', 'Enabled'}  vector_style=Wide Row  use_help_units=on  help='Liquid fuel rate based on airflow and target equivalence ratio'  units='g/s'  use_header_enum=off  row_header_enum={}  col_header_enum={}  use_precision=off  precision=''  gain=1  offset=0  exp=1  use_mototune_group=on  mototune_group=motohawk_vardec_path(gcb)
  motohawk_probe1 : MotoHawk_lib/Calibration & Probing Blocks/motohawk_probe  nam='PerCylBaseFuelRate'  show_more=on  name_source=Use Parameter  read_level=1  view_as=Number  enum_struct={'Disabled', 'Enabled'}  vector_style=Wide Row  use_help_units=on  help='Liquid fuel mass flow rate based on airflow and target equivalence ratio per cylinder.'  units='g/s'  use_header_enum=off  row_header_enum={}  col_header_enum={}  use_precision=off  precision=''  gain=1  offset=0  exp=1  use_mototune_group=on  mototune_group=motohawk_vardec_path(gcb)
  motohawk_probe2 : MotoHawk_lib/Calibration & Probing Blocks/motohawk_probe  nam='AdjustedPerCylFuelRate'  show_more=on  name_source=Use Parameter  read_level=1  view_as=Number  enum_struct={'Disabled', 'Enabled'}  vector_style=Wide Row  use_help_units=on  help='Desired fuel per cylinder after application of individual cylinder offsets and multipliers.'  units='g/s'  use_header_enum=off  row_header_enum={}  col_header_enum={}  use_precision=off  precision=''  gain=1  offset=0  exp=1  use_mototune_group=on  mototune_group=motohawk_vardec_path(gcb)
  Fuel : Outport
  wires:
  "Apply Multipliers for O2, Knock Control, and Enrichment1"/1 -> Fuel/1, motohawk_probe2/1
  O2Info/1 -> Bus Selector1/1, Bus Selector/1
  Data Type Conversion/1 -> Per-Cylinder Mass Flow Rate/2
  Number of Combustion Events Per Revolution/1 -> Data Type Conversion/1
  Calculate Fuel Flow/1(BaseFuelRate [g/s]) -> Per-Cylinder Mass Flow Rate/1, motohawk_probe/1
  Per-Cylinder Mass Flow Rate/1 -> motohawk_probe1/1, "Apply Multipliers for O2, Knock Control, and Enrichment1"/1
  Sensors/1 -> Calculate Fuel Flow/2(Sensors)
  Bus Selector1/1 -> Calculate Fuel Flow/1(DesEquivRatio)  "<DesEquivRatio>"
  Bus Selector/1 -> "Apply Multipliers for O2, Knock Control, and Enrichment1"/2  "<O2FuelMult>"

== system BaseEngineController_LS_128/Foreground/Control/Controller/Run/Fuel System Manager/Injector Manager ==
  Fuel : Inport
  Sensors : Inport  Port=2
  Bus Selector : BusSelector  OutputSignals=RawIndexes.MAP09Idx
  Bus Selector1 : BusSelector  OutputSignals=RawIndexes.RPM09Idx
  Bus Selector2 : BusSelector  OutputSignals=Raw.RPM
  Bus Selector4 : BusSelector  OutputSignals=RawProcessed.TPS,AirCalcs.MAFPort,RawIndexes.ECT05Idx,Raw.LinearSensors.MAP_Angular,RawIndexes.OXY05Idx
  Constant1 : Constant  OutDataTypeStr=Inherit: Inherit via back propagation
  Delta TPS Transient Fueling : Subsystem  TreatAsAtomicUnit=on
      mask Display:
      | patch([0 0 1 1], [0 0.075 0.075 0], [230/255 0/255 0/255])
      | patch([0 0 1 1], [0.025 0.05 0.05 0.025], [150/255 0/255 0/255])
      | patch([0 0 1 1], [0 0.025 0.025 0], [0/255 0/255 0/255])
      | 
      | disp('TRANSIENT\nFUELING\nMULTIPLIER')
  Divide : Product  Inputs=**
  Make-Up Pulse End of Injection Timing1 : MotoHawk_lib/Lookup Tables/motohawk_interpolation_2d  nam='MakeUpEOI'  table_data=ones(9)*200  show_more=on  data_type=Inherit from 'Table Data'  storage=NonAdaptive  read_level=1  write_level=1  ovr_cals=on  use_help=on  help='End of injection timing for transient makeup fuel pulse'  units='degBTDC'  use_min_max=on  min_val=-1000  max_val=1000  use_precision=on  precision=''  gain=1  offset=0  exp=1  use_links=off  row_prelookup_block=''  col_prelookup_block=''  output_name=''  use_mototune_group=on  mototune_group=motohawk_vardec_path(gcb)
  Mass Flow to Charge Mass Transform : motohawk_engine_lib/Mass Flow to Charge Mass Transform  SystemSampleTime=-1
  Primary Pulse Injection Timing : MotoHawk_lib/Lookup Tables/motohawk_interpolation_2d  nam='PrimarySOI'  table_data=ones(9)*600  show_more=on  data_type=Inherit from 'Table Data'  storage=NonAdaptive  read_level=1  write_level=1  ovr_cals=on  use_help=on  help='Injection timing for primary fuel pulse - SOI or EOI depending on Inj Config'  units='degBTDC'  use_min_max=on  min_val=-1000  max_val=1000  use_precision=on  precision=''  gain=1  offset=0  exp=1  use_links=off  row_prelookup_block=''  col_prelookup_block=''  output_name=''  use_mototune_group=on  mototune_group=motohawk_vardec_path(gcb)
  motohawk_calibration1 : MotoHawk_lib/Calibration & Probing Blocks/motohawk_calibration  nam='DeltaTPSFuelingEnable'  val=1  storage=Calibration  show_more=on  name_source=Use Parameter  data_type=boolean  read_level=1  write_level=1  ovr_cals=on  view_as=Enumeration  enum_struct={'Disabled', 'Enabled'}  vector_style=Wide Row  use_help_units=on  help='Enable Delta TPS transient fuel algorithm'  units=''  use_header_enum=off  row_header_enum={}  col_header_enum={}  use_min_max=off  min_val=-inf  max_val=inf  use_precision=off  precision=''  gain=1  offset=0  exp=1  use_mototune_group=on  mototune_group=motohawk_vardec_path(gcb)
  PrimaryInjTiming : Outport
  MakeUpInjTiming : Outport  Port=2
  FPC : Outport  Port=3
  wires:
  Sensors/1 -> Bus Selector1/1, Bus Selector/1, Bus Selector2/1, Bus Selector4/1
  Bus Selector/1 -> Primary Pulse Injection Timing/1, Make-Up Pulse End of Injection Timing1/1  "<MAP09Idx>"
  Bus Selector1/1 -> Primary Pulse Injection Timing/2, Make-Up Pulse End of Injection Timing1/2  "<RPM09Idx>"
  Bus Selector2/1 -> Mass Flow to Charge Mass Transform/2  "<RPM>"
  Mass Flow to Charge Mass Transform/1 -> FPC/1
  Bus Selector4/1 -> Delta TPS Transient Fueling/1(TPS)  "<TPS>"
  Bus Selector4/2 -> Delta TPS Transient Fueling/2(MAF)  "<MAFPort>"
  Bus Selector4/3 -> Delta TPS Transient Fueling/3(ECTIdx)  "<ECT05Idx>"
  Fuel/1 -> Divide/2
  Delta TPS Transient Fueling/1(DeltaTPSMult) -> Divide/1
  Divide/1 -> Mass Flow to Charge Mass Transform/1
  motohawk_calibration1/1 -> Delta TPS Transient Fueling/Enable
  Primary Pulse Injection Timing/1 -> PrimaryInjTiming/1
  Make-Up Pulse End of Injection Timing1/1 -> MakeUpInjTiming/1  "EOI"
  Bus Selector4/4 -> Delta TPS Transient Fueling/4(MAPAngle)  "<MAP_Angular>"
  Bus Selector4/5 -> Delta TPS Transient Fueling/5(OxyIdx)  "<OXY05Idx>"
  Constant1/1 -> Mass Flow to Charge Mass Transform/3
